simulink model "if_2"  (R2021a)
settings: Solver=FixedStepAuto  StartTime=0.0  StopTime=10.0  FixedStep=1e-3  RelTol=1e-3
libraries: simulink x1
settings Model: Creator=yasso  LastModifiedBy=yasso

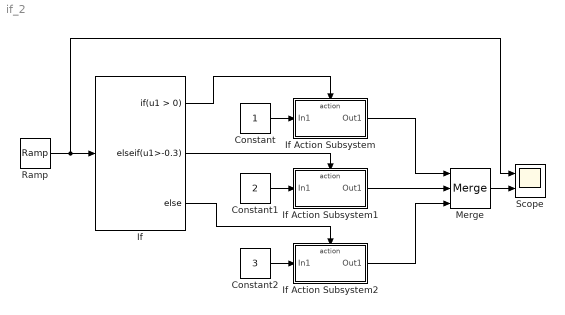
== system if_2 ==
  Constant : Constant
  Constant1 : Constant  Value=2
  Constant2 : Constant  Value=3
  If : If  ElseIfExpressions=u1>-0.3
  If Action Subsystem : Subsystem  TreatAsAtomicUnit=on
  If Action Subsystem1 : Subsystem  TreatAsAtomicUnit=on
  If Action Subsystem2 : Subsystem  TreatAsAtomicUnit=on
  Merge : Merge  Inputs=3
  Ramp : simulink/Sources/Ramp  slope=1  start=0  InitialOutput=-3
  Scope : Scope  NumInputPorts=2
  wires:
  If/1 -> If Action Subsystem/Action
  Constant/1 -> If Action Subsystem/1(In1)
  If/2 -> If Action Subsystem1/Action
  Constant1/1 -> If Action Subsystem1/1(In1)
  If/3 -> If Action Subsystem2/Action
  Constant2/1 -> If Action Subsystem2/1(In1)
  If Action Subsystem2/1(Out1) -> Merge/3
  If Action Subsystem1/1(Out1) -> Merge/2
  If Action Subsystem/1(Out1) -> Merge/1
  Ramp/1 -> Scope/1, If/1
  Merge/1 -> Scope/2

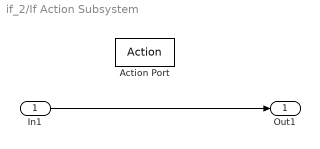
== system if_2/If Action Subsystem ==
  In1 : Inport
  Action Port : ActionPort  ActionPortLabel=if(u1 > 0)
  Out1 : Outport
  wires:
  In1/1 -> Out1/1

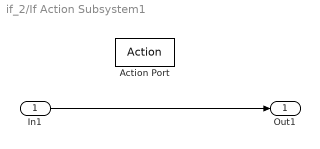
== system if_2/If Action Subsystem1 ==
  In1 : Inport
  Action Port : ActionPort  ActionPortLabel=elseif(u1>-0.3)
  Out1 : Outport
  wires:
  In1/1 -> Out1/1

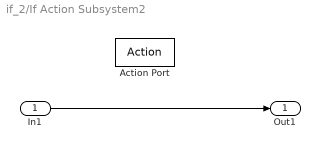
== system if_2/If Action Subsystem2 ==
  In1 : Inport
  Action Port : ActionPort  ActionPortLabel=else
  Out1 : Outport
  wires:
  In1/1 -> Out1/1
